simulink model "Optitrack_Visualization_r2018a"  (Simulink 9.1)
settings: Solver=FixedStepDiscrete  StartTime=0.0  StopTime=inf  FixedStep=0.001  RelTol=1e-3  EnableMultiTasking=on
undefined symbols (not defined in the file): qc_get_step_size
libraries: quarc_library x6
settings Model: Creator=glai  LastModifiedBy=user  SimulationMode=external  ExtModeTrigDuration=5000
settings SolverCC: PositivePriorityOrder=on
settings DataIOCC: LimitDataPoints=on
settings OptimizationCC: LifeSpan=auto
settings DebuggingCC: UnderspecifiedInitializationDetection=Simplified  MergeDetectMultiDrivingBlocksExec=error  SolverPrmCheckMsg=warning
settings HardwareCC: ProdBitPerPointer=64  ProdBitPerSizeT=64  ProdBitPerPtrDiffT=64  ProdLargestAtomicFloat=Float  ProdIntDivRoundTo=Zero  ProdEndianess=LittleEndian  ProdWordSize=64  ProdHWDeviceType=Intel->x86-64 (Windows64)
settings RTWCC: Description=QUARC Win64 Target Using Toolchain  SystemTargetFile=quarc_win64.tlc  TemplateMakefile=quarc_default_tmf  Toolchain=QUARC win64 | nmake (64-bit Windows)  BuildConfiguration=Faster Runs
settings STFCustomTargetCC: ConcurrentExecutionCompliant=on  UseToolchainInfoCompliant=on  SystemTargetFile=quarc_win64.tlc
settings GRTTargetCC: ParMdlRefBuildCompliant=off  CompOptLevelCompliant=off  MatFileLogging=off  CPPClassGenCompliant=off  ExtMode=on  ExtModeMexFile=quarc_comm  ExtModeMexArgs='-w -d %d -uri %u', 'shmem://%m:1?timeout=10'
settings ConfigComp: CovSFcnEnable=off

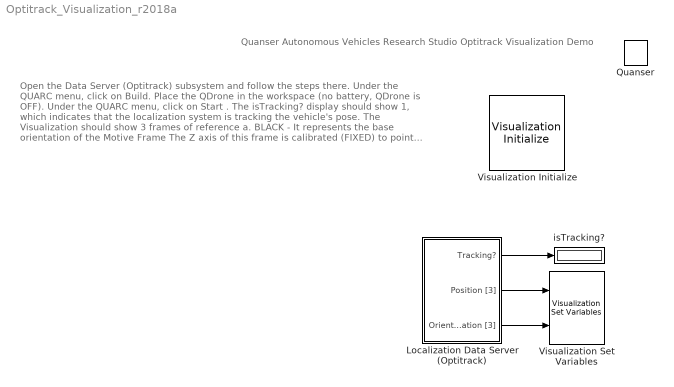
== system Optitrack_Visualization_r2018a ==
  note: Quanser Autonomous Vehicles Research Studio
      | Optitrack Visualization Demo
  note: Open the Data Server (Optitrack) subsystem and follow the steps there.
      |
      | Under the QUARC menu, click on Build.
      |
      | Place the QDrone in the workspace (no battery, QDrone is OFF).
      |
      | Under the QUARC menu, click on Start .
      |
      | The isTracking? display should show 1, which indicates that the localization system is tracking the vehicle's pose.
      |
      | The Visualization should show 3 frames of reference
      | a. BLACK - It represents the base orientation of the Motive Frame
      | The Z axis of this frame is calibrated (FIXED) to point towards the
      | ground control station PC.
      |
      | b. BLUE - It represents the base orientation Research Studio Frame
      | which is FIXED in space and it's origin aligns with Motive Frame.
      | The X axis of the Research Studio Frame (also the direction of 0 heading/yaw)
      | points away from the ground control station PC (directly opposite to the Z axis
      | of the Motive Frame).
      |
      | c. RED - It represents the position and orientation of the QDrone's Body-Fixed Reference Frame as measured by OptiTrack data directly.
      |
      | When the vehicle is located at the workspace origin with 0 orientation (i.e., 0 Roll, 0 Pitch and 0 Yaw), the vehicle Body-Fixed Reference Frame will align with the Research Studio Frame (BLUE Basis Arrows).
      |
      | Step into the workspace and move the QDrone around by hand. The RED frame should move as it is Body-Fixed w.r.t. the QDrone.
      | NOTE : Hold the QDrone using the handle provided on the top frame
      |
      | Stop the model when finished.
  "Localization Data Server (Optitrack) " : Subsystem
  Quanser : quarc_library/Logos/Quanser
  Visualization Initialize : quarc_library/User Interface/Visualization/Visualization Initialize  object_name=POSE_Check  scene_file=POSE_Check.xml  uri={'normal','';'Configuration','shmem://%m:2';}  apply_uri_to_all_configs=off  server_send_size=1000000  server_receive_size=1000  derive_from_server=on  client_send_size=1000  client_receive_size=1000000  variables=[ 60 61 80 81 ]  initial_values=single([ 0 0 0 0 0 0 0 0 0 0 0 0 ])  open_on_start=on  close_on_stop=on
      settings: AttributesFormatString=%<object_name>  SourceProductName=QUARC Targets
  Visualization Set Variables : quarc_library/User Interface/Visualization/Visualization Set Variables  object_name=POSE_Check  offset=[ 0 0 ]  data_type=[ 0 0 ]  length=[ 1 1 ]  sample_time=visualization_get_frame_period  actor_name={'actor.RefFrame.BodyFixed.OptiTrack/Position';'actor.RefFrame.BodyFixed.OptiTrack/Orientation'}
      settings: AttributesFormatString=(%<object_name>)  SourceProductName=QUARC Targets
  isTracking? : Display
  wires:
  "Localization Data Server (Optitrack) "/2(Position [3]) -> Visualization Set Variables/1
  "Localization Data Server (Optitrack) "/3(Orientation [3]) -> Visualization Set Variables/2
  "Localization Data Server (Optitrack) "/1(Tracking?) -> isTracking?/1

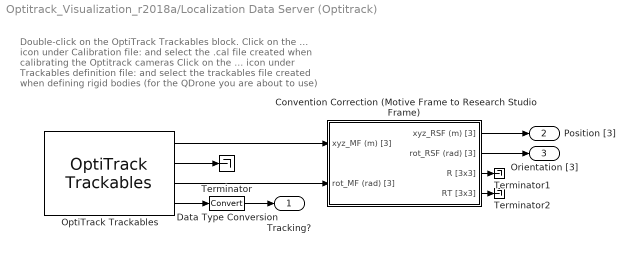
== system Optitrack_Visualization_r2018a/Localization Data Server (Optitrack)  ==
  note: Double-click on the OptiTrack Trackables block.
      |
      | Click on the ... icon under Calibration file: and select the .cal file
      | created when calibrating the Optitrack cameras
      |
      | Click on the ... icon under Trackables definition file: and select
      | the trackables file created when defining rigid bodies (for the
      | QDrone you are about to use)
  Convention Correction (Motive Frame to Research Studio Frame) : Subsystem
  Data Type Conversion : DataTypeConversion
  OptiTrack Trackables : quarc_library/Devices/Third-Party/NaturalPoint/OptiTrack/OptiTrack Trackables  calibration_file=C:\Users\user\Documents\OptiTrack\Session 2018-05-08\Calibration Exceptional (MeanErr 0.536 mm) 2018-05-08 10.cal  rigid_body_file=C:\Users\user\Documents\OptiTrack\Session 2018-05-08\Qdrone038682.tra  rigid_body_ids=[1]  sample_time=qc_get_step_size*10  active=off
      settings: SourceProductName=QUARC Targets
  Terminator : Terminator
  Terminator1 : Terminator
  Terminator2 : Terminator
  Tracking? : Outport  VectorParamsAs1DForOutWhenUnconnected=off
  Position [3] : Outport  Port=2  VectorParamsAs1DForOutWhenUnconnected=off
  Orientation [3] : Outport  Port=3  VectorParamsAs1DForOutWhenUnconnected=off
  wires:
  OptiTrack Trackables/2 -> Terminator/1
  OptiTrack Trackables/4 -> Data Type Conversion/1
  Data Type Conversion/1 -> Tracking?/1
  OptiTrack Trackables/1 -> Convention Correction (Motive Frame to Research Studio Frame)/1(xyz_MF (m) [3])
  OptiTrack Trackables/3 -> Convention Correction (Motive Frame to Research Studio Frame)/2(rot_MF (rad) [3])
  Convention Correction (Motive Frame to Research Studio Frame)/1(xyz_RSF (m) [3]) -> Position [3]/1
  Convention Correction (Motive Frame to Research Studio Frame)/2(rot_RSF (rad) [3]) -> Orientation [3]/1
  Convention Correction (Motive Frame to Research Studio Frame)/3(R [3x3]) -> Terminator1/1
  Convention Correction (Motive Frame to Research Studio Frame)/4(RT [3x3]) -> Terminator2/1

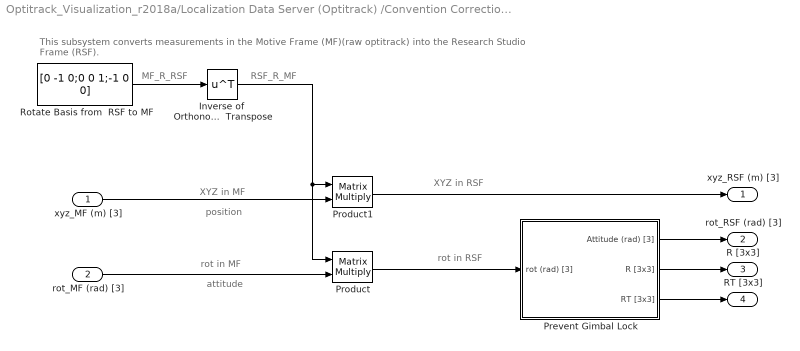
== system Optitrack_Visualization_r2018a/Localization Data Server (Optitrack) /Convention Correction (Motive Frame to Research Studio Frame) ==
  note: MF_R_RSF
  note: This subsystem converts measurements in the Motive Frame (MF)(raw optitrack) into the Research Studio Frame (RSF).
  note: RSF_R_MF
  note: XYZ in MF
  note: rot in MF
  note: position
  note: attitude
  note: XYZ in RSF
  note: rot in RSF
  xyz_MF (m) [3] : Inport
  rot_MF (rad) [3] : Inport  Port=2
  Inverse of  Orthonormal  Matrix is its  Transpose : Math  Operator=transpose  SaturateOnIntegerOverflow=on
  Prevent Gimbal Lock : Subsystem
  Product : Product  Multiplication=Matrix(*)
  Product1 : Product  Multiplication=Matrix(*)
  Rotate Basis from  RSF to MF : Constant  Value=[0 -1 0;0 0 1;-1 0 0]
  xyz_RSF (m) [3] : Outport  VectorParamsAs1DForOutWhenUnconnected=off
  rot_RSF (rad) [3] : Outport  Port=2  VectorParamsAs1DForOutWhenUnconnected=off
  R [3x3] : Outport  Port=3  VectorParamsAs1DForOutWhenUnconnected=off
  RT [3x3] : Outport  Port=4  VectorParamsAs1DForOutWhenUnconnected=off
  wires:
  Rotate Basis from  RSF to MF/1 -> Inverse of  Orthonormal  Matrix is its  Transpose/1
  xyz_MF (m) [3]/1 -> Product1/2
  Inverse of  Orthonormal  Matrix is its  Transpose/1 -> Product1/1, Product/1
  rot_MF (rad) [3]/1 -> Product/2
  Product1/1 -> xyz_RSF (m) [3]/1
  Product/1 -> Prevent Gimbal Lock/1(rot (rad) [3])
  Prevent Gimbal Lock/1(Attitude (rad) [3]) -> rot_RSF (rad) [3]/1
  Prevent Gimbal Lock/2(R [3x3]) -> R [3x3]/1
  Prevent Gimbal Lock/3(RT [3x3]) -> RT [3x3]/1

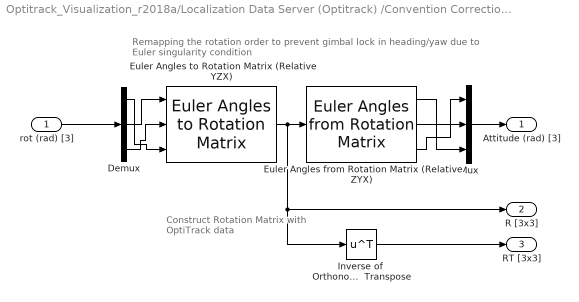
== system Optitrack_Visualization_r2018a/Localization Data Server (Optitrack) /Convention Correction (Motive Frame to Research Studio Frame)/Prevent Gimbal Lock ==
  note: Construct Rotation Matrix
      | with OptiTrack data
  note: Remapping the rotation order to prevent gimbal lock
      | in heading/yaw due to Euler singularity condition
  rot (rad) [3] : Inport
  Demux : Demux  Outputs=3
  Euler Angles from Rotation Matrix (Relative ZYX) : quarc_library/Math Operations/Matrices/Euler Angles from Rotation Matrix  menu_order=Relative Z-Y-X
      settings: SourceProductName=QUARC Targets
  Euler Angles to Rotation Matrix (Relative YZX) : quarc_library/Math Operations/Matrices/Euler Angles to Rotation Matrix  menu_order=Relative Y-Z-X
      settings: SourceProductName=QUARC Targets
  Inverse of  Orthonormal  Matrix is its  Transpose : Math  Operator=transpose  SaturateOnIntegerOverflow=on
  Mux : Mux  Inputs=3
  Attitude (rad) [3] : Outport  VectorParamsAs1DForOutWhenUnconnected=off
  R [3x3] : Outport  Port=2  VectorParamsAs1DForOutWhenUnconnected=off
  RT [3x3] : Outport  Port=3  VectorParamsAs1DForOutWhenUnconnected=off
  wires:
  Euler Angles from Rotation Matrix (Relative ZYX)/2 -> Mux/2
  Euler Angles from Rotation Matrix (Relative ZYX)/1 -> Mux/3
  Euler Angles from Rotation Matrix (Relative ZYX)/3 -> Mux/1
  Euler Angles to Rotation Matrix (Relative YZX)/1 -> R [3x3]/1, Inverse of  Orthonormal  Matrix is its  Transpose/1, Euler Angles from Rotation Matrix (Relative ZYX)/1
  rot (rad) [3]/1 -> Demux/1
  Mux/1 -> Attitude (rad) [3]/1
  Demux/2 -> Euler Angles to Rotation Matrix (Relative YZX)/1
  Demux/3 -> Euler Angles to Rotation Matrix (Relative YZX)/2
  Demux/1 -> Euler Angles to Rotation Matrix (Relative YZX)/3
  Inverse of  Orthonormal  Matrix is its  Transpose/1 -> RT [3x3]/1
